simulink library "EV_ePWT"  (R2019b)
settings: Solver=VariableStepAuto  StartTime=0.0  StopTime=10.0  RelTol=1e-3
undefined symbols (not defined in the file): BTR, DiscIntNeverNeededParam, INV
libraries: simulink x1
(part 2 of 2)

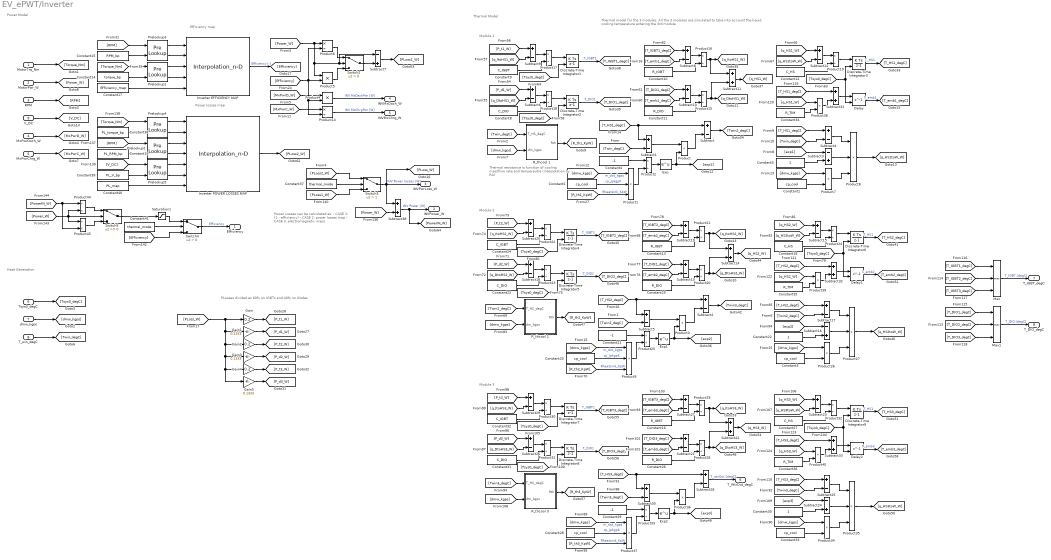
== system EV_ePWT/Inverter ==
  note: Efficiency map
  note: Module 1
  note: Heat Generation
  note: Power Model
  note: Thermal Model
  note: Module 2
  note: Module 3
  note: Power Losses can be calculated as:
      | - CASE 1: (1 - efficiency)
      | - CASE 2: power losses map
      | - CASE 3: electromagnetic maps
  note: PLosses divided as 60% on IGBTs and 40% on diodes
  note: Thermal model for the 3 modules. All the 3 modules are simulated to take into account the liquid cooling temperature entering the 3rd module
  note: Thermal resistance is function of cooling massflow rate and temperautre (interpolation by RA)
  note: Power losses map
  MotorTrq_Nm : Inport
  MotorPwr_W : Inport  Port=2
  RPM : Inport  Port=3
  MxPwrDsch_W : Inport  Port=4
  MxPwrChrg_W : Inport  Port=5
  Tsys0_degC : Inport  Port=6
  dmw_kgps : Inport  Port=7
  T_win_degC : Inport  Port=8
  V_DC : Inport  Port=9
  Constant{1..3,20,28,33} (6 alike) : Constant  Value=cp_cool
  Constant10 : Constant  Value=R_IGBT
  Constant11 : Constant  Value=R_DIO
  Constant12 : Constant  Value=C_HS
  Constant13 : Constant  Value=R_IGBT
  Constant14 : Constant  Value=torque_bp
  Constant15 : Constant  Value=RPM_bp
  Constant16 : Constant  Value=R_IGBT
  Constant17 : Constant  Value=Efficiency_map
  Constant18 : Constant  Value=C_HS
  Constant19 : Constant  Value=PL_RPM_bp
  Constant21 : Constant  Value=-1
  Constant22 : Constant
  Constant23 : Constant  Value=C_DIO
  Constant24 : Constant  Value=C_IGBT
  Constant25 : Constant  Value=R_DIO
  Constant26 : Constant  Value=R_DIO
  Constant27 : Constant  Value=C_HS
  Constant29 : Constant  Value=-1
  Constant30 : Constant
  Constant31 : Constant  Value=C_DIO
  Constant32 : Constant  Value=C_IGBT
  Constant34 : Constant  Value=R_TIM
  Constant35 : Constant  Value=R_TIM
  Constant36 : Constant  Value=R_TIM
  Constant37 : Constant  Value=thermal_mode
  Constant38 : Constant  Value=PL_torque_bp
  Constant39 : Constant  Value=PL_V_bp
  Constant4 : Constant  Value=-1
  Constant40 : Constant  Value=PL_map
  Constant41 : Constant  Value=thermal_mode
  Constant5 : Constant
  Constant8 : Constant  Value=C_DIO
  Constant9 : Constant  Value=C_IGBT
  Delay : Delay  DelayLength=1  InitialConditionSource=Input port
      settings: InputPortMap=u0,p4
  Delay1 : Delay  DelayLength=1  InitialConditionSource=Input port
      settings: InputPortMap=u0,p4
  Delay2 : Delay  DelayLength=1  InitialConditionSource=Input port
      settings: InputPortMap=u0,p4
  Discrete-Time Integrator{1..9} (9 alike) : DiscreteIntegrator  InitialConditionSource=external  SampleTime=-1  ICPrevOutput=DiscIntNeverNeededParam  ICPrevScaledInput=DiscIntNeverNeededParam
  Exp : Math  SaturateOnIntegerOverflow=on
  Exp1 : Math  SaturateOnIntegerOverflow=on
  Exp2 : Math  SaturateOnIntegerOverflow=on
  Gain : Gain  Gain=0.2
  Gain1 : Gain  Gain=0.1333
  Gain2 : Gain  Gain=0.2
  Gain3 : Gain  Gain=0.1333
  Gain4 : Gain  Gain=0.2
  Gain5 : Gain  Gain=0.1333
  Inverter EFFICIENCY MAP : Interpolation_n-D  TableSource=Input port
      settings: InputPortMap=u0,u1,u2,u3,p2
  Inverter POWER LOSSES MAP : Interpolation_n-D  NumberOfTableDimensions=3  TableSource=Input port
      settings: InputPortMap=u0,u1,u2,u3,u4,u5,p2
  Max : MinMax  Function=max  Inputs=3
  Max1 : MinMax  Function=max  Inputs=3
  Prelookup{1..5} (5 alike) : PreLookup  BreakpointsDataSource=Input port  BreakpointsData=[1:4]  ExtrapMethod=Linear  FractionDataTypeStr=double
      settings: InputPortMap=u0,p1
  Product{,3..5,7,26,34,36} (8 alike) : Product
  Product{1,8..9,27,35,37} (6 alike) : Product  Inputs=3
  Product{2,6,14..25,28..33} (20 alike) : Product  Inputs=*/
  Product38 : Product  Inputs=**
  Product39 : Product  Inputs=**
  Product40 : Product  Inputs=**
  Product44 : Product  Inputs=/*
  Product45 : Product  Inputs=/*
  R_thcool 1 : MATLAB Function  TreatAsAtomicUnit=on
  R_thcool 2 : MATLAB Function  TreatAsAtomicUnit=on
  R_thcool 3 : MATLAB Function  TreatAsAtomicUnit=on
  Saturation1 : Saturate  UpperLimit=1  LowerLimit=0.25
  Subtract{,1..2,4..6,8..10,12..13,15,17..21,23,25..30} (24 alike) : Sum  Inputs=+-
  Subtract{11,14,22,31..33,38} (7 alike) : Sum
  Subtract{3,7,16,24} (4 alike) : Sum  Inputs=-+
  Switch2 : Switch  Criteria=u2 > Threshold
  Switch3 : Switch  Criteria=u2 > Threshold  Threshold=1
  Switch4 : Switch  Criteria=u2 > Threshold
  Switch5 : Switch
  Efficiency : Outport
  INVPower_W : Outport  Port=2
  INVPwrLoss_W : Outport  Port=3
  INVMxDsch_W : Outport  Port=4
  INVMxChrg_W : Outport  Port=5
  T_WtrOut_degC : Outport  Port=6
  T_IGBT_degC : Outport  Port=7
  T_DIO_degC : Outport  Port=8
  wires:
  Delay2/1 -> [T_emb3_degC]  "T_emb3"
  Subtract33/1 -> Delay2/1
  Product40/1 -> Subtract33/2
  [T_HS3_degC] -> Subtract33/1
  Constant36/1 -> Product40/2
  [q_HS3_W] -> Product40/1
  [Tsys0_degC] -> Discrete-Time Integrator9/2, Delay2/2
  [Tsys0_degC] -> Discrete-Time Integrator6/2, Delay1/2
  [q_HS2_W] -> Product39/1
  Constant35/1 -> Product39/2
  [T_HS2_degC] -> Subtract32/1
  Product39/1 -> Subtract32/2
  Subtract32/1 -> Delay1/1
  Delay1/1 -> [T_emb2_degC]  "T_emb2"
  Delay/1 -> [T_emb1_degC]  "T_emb1"
  Subtract31/1 -> Delay/1
  Product38/1 -> Subtract31/2
  [T_HS1_degC] -> Subtract31/1
  Constant34/1 -> Product38/2
  [q_HS1_W] -> Product38/1
  R_thcool 1/1(Rth) -> [R_th1_KpW]
  T_win_degC/1 -> [Twin_degC]
  dmw_kgps/1 -> [dmw_kgps]
  Product6/1 -> Switch2/1
  [Efficiency] -> Product5/2, Product6/2, Product14/2, Product4/2
  [RPM] -> Prelookup3/1
  Prelookup3/1 -> Inverter EFFICIENCY MAP/1
  Prelookup3/2 -> Inverter EFFICIENCY MAP/2
  Constant15/1 -> Prelookup3/2
  Inverter EFFICIENCY MAP/1 -> [Efficiency]  "Efficiency [-]"
  MotorTrq_Nm/1 -> [Torque_Nm]
  Tsys0_degC/1 -> [Tsys0_degC]
  MxPwrDsch_W/1 -> [MxPwrD_W]
  RPM/1 -> [RPM]
  MxPwrChrg_W/1 -> [MxPwrC_W]
  MotorPwr_W/1 -> [Power_W]
  [Power_W] -> Subtract7/1, Switch2/2, Product5/1, Product6/1
  [MxPwrD_W] -> Product4/1
  Product4/1 -> INVMxDsch_W/1  "INV MxDschPwr [W]"
  Product14/1 -> INVMxChrg_W/1  "INV MxChrgPwr [W]"
  [MxPwrC_W] -> Product14/1
  Subtract4/1 -> Product8/1
  Product8/1 -> [q_HS1toW_W]
  [dmw_kgps] -> Product1/1  "m_dot_kgps"
  Product7/1 -> Product8/3
  Subtract1/1 -> Product/1
  [T_HS1_degC] -> Subtract4/1
  [dmw_kgps] -> Product7/1
  [Twin_degC] -> Subtract4/2
  Subtract3/1 -> Product8/2
  Product/1 -> Subtract/2
  Exp/1 -> [exp1], Product/2
  Constant2/1 -> Product1/2  "cp_JpkgpK"
  Constant1/1 -> Product7/2
  [R_th1_KpW] -> Product1/3  "Rheatsink_KpW"
  Product2/1 -> Exp/1
  Product1/1 -> Product2/2
  Constant4/1 -> Product2/1
  [Twin_degC] -> Subtract1/2
  [T_HS1_degC] -> Subtract1/1, Subtract/1
  [exp1] -> Subtract3/1
  Constant5/1 -> Subtract3/2
  V_DC/1 -> [V_DC]
  Subtract9/1 -> Product17/1
  [q_DtoHS1_W] -> Subtract6/2
  Discrete-Time Integrator1/1 -> [T_IGBT1_degC]  "T_IGBT1"
  Constant8/1 -> Product18/2
  Subtract6/1 -> Product18/1
  Product18/1 -> Discrete-Time Integrator2/1
  [Tsys0_degC] -> Discrete-Time Integrator2/2
  [P_t1_W] -> Subtract9/1
  Subtract11/1 -> [q_HS1_W]
  [P_d1_W] -> Subtract6/1
  Product17/1 -> Discrete-Time Integrator1/1
  Discrete-Time Integrator2/1 -> [T_DIO1_degC]  "T_DIO1"
  [Tsys0_degC] -> Discrete-Time Integrator1/2
  [q_ItoHS1_W] -> Subtract9/2
  Constant9/1 -> Product17/2
  Subtract8/1 -> Product16/1
  [T_IGBT1_degC] -> Subtract8/1
  [T_emb1_degC] -> Subtract8/2
  Constant10/1 -> Product16/2
  Constant11/1 -> Product15/2
  [T_emb1_degC] -> Subtract10/2
  [T_DIO1_degC] -> Subtract10/1
  Subtract10/1 -> Product15/1
  Product16/1 -> Subtract11/1, [q_ItoHS1_W]
  Product15/1 -> Subtract11/2, [q_DtoHS1_W]
  Constant12/1 -> Product19/2
  [Tsys0_degC] -> Discrete-Time Integrator3/2, Delay/2
  Product19/1 -> Discrete-Time Integrator3/1
  Subtract12/1 -> Product19/1
  [q_HS1_W] -> Subtract12/1
  [q_HS1toW_W] -> Subtract12/2
  Discrete-Time Integrator3/1 -> [T_HS1_degC]  "T_HS1"
  [Twin_degC] -> R_thcool 1/1(T_HS_degC)
  [dmw_kgps] -> R_thcool 1/2(dm_kgps)
  Subtract/1 -> [Twin2_degC]
  Subtract2/1 -> [Twin3_degC]
  R_thcool 2/1(Rth) -> [R_th2_KpW]
  [dmw_kgps] -> R_thcool 2/2(dm_kgps)
  [Twin2_degC] -> R_thcool 2/1(T_HS_degC)
  Discrete-Time Integrator6/1 -> [T_HS2_degC]  "T_HS1"
  [q_HS2toW_W] -> Subtract15/2
  [q_HS2_W] -> Subtract15/1
  Subtract15/1 -> Product24/1
  Product24/1 -> Discrete-Time Integrator6/1
  Constant18/1 -> Product24/2
  Product20/1 -> [q_DtoHS2_W], Subtract14/2
  Product21/1 -> [q_ItoHS2_W], Subtract14/1
  Subtract13/1 -> Product20/1
  [T_DIO2_degC] -> Subtract13/1
  [T_emb2_degC] -> Subtract13/2
  Constant25/1 -> Product20/2
  Constant13/1 -> Product21/2
  [T_emb2_degC] -> Subtract19/2
  [T_IGBT2_degC] -> Subtract19/1
  Subtract19/1 -> Product21/1
  Constant24/1 -> Product22/2
  [q_ItoHS2_W] -> Subtract20/2
  [Tsys0_degC] -> Discrete-Time Integrator4/2
  Discrete-Time Integrator5/1 -> [T_DIO2_degC]  "T_DIO1"
  Product22/1 -> Discrete-Time Integrator4/1
  [P_d2_W] -> Subtract18/1
  Subtract14/1 -> [q_HS2_W]
  [P_t2_W] -> Subtract20/1
  [Tsys0_degC] -> Discrete-Time Integrator5/2
  Product23/1 -> Discrete-Time Integrator5/1
  Subtract18/1 -> Product23/1
  Constant23/1 -> Product23/2
  Discrete-Time Integrator4/1 -> [T_IGBT2_degC]  "T_IGBT1"
  [q_DtoHS2_W] -> Subtract18/2
  Subtract20/1 -> Product22/1
  Constant22/1 -> Subtract16/2
  [exp2] -> Subtract16/1
  [T_HS2_degC] -> Subtract2/1, Subtract5/1
  [Twin2_degC] -> Subtract5/2
  Constant21/1 -> Product25/1
  Product9/1 -> Product25/2
  Product25/1 -> Exp1/1
  [R_th2_KpW] -> Product9/3  "Rheatsink_KpW"
  Constant3/1 -> Product26/2
  Constant20/1 -> Product9/2  "cp_JpkgpK"
  Exp1/1 -> Product3/2, [exp2]
  Product3/1 -> Subtract2/2
  Subtract16/1 -> Product27/2
  [Twin2_degC] -> Subtract17/2
  [dmw_kgps] -> Product26/1
  [T_HS2_degC] -> Subtract17/1
  Subtract5/1 -> Product3/1
  Product26/1 -> Product27/3
  [dmw_kgps] -> Product9/1  "m_dot_kgps"
  Product27/1 -> [q_HS2toW_W]
  Subtract17/1 -> Product27/1
  Subtract25/1 -> Product35/1
  Product35/1 -> [q_HS3toW_W]
  [dmw_kgps] -> Product37/1  "m_dot_kgps"
  Product34/1 -> Product35/3
  Subtract30/1 -> Product36/1
  [T_HS3_degC] -> Subtract25/1
  [dmw_kgps] -> Product34/1
  [Twin3_degC] -> Subtract25/2
  Subtract24/1 -> Product35/2
  Product36/1 -> Subtract28/2
  Exp2/1 -> [exp3], Product36/2
  Constant28/1 -> Product37/2  "cp_JpkgpK"
  Constant33/1 -> Product34/2
  [R_th3_KpW] -> Product37/3  "Rheatsink_KpW"
  Product33/1 -> Exp2/1
  Product37/1 -> Product33/2
  Constant29/1 -> Product33/1
  [Twin3_degC] -> Subtract30/2
  [T_HS3_degC] -> Subtract30/1, Subtract28/1
  [exp3] -> Subtract24/1
  Constant30/1 -> Subtract24/2
  Subtract29/1 -> Product30/1
  [q_DtoHS3_W] -> Subtract26/2
  Discrete-Time Integrator7/1 -> [T_IGBT3_degC]  "T_IGBT1"
  Constant31/1 -> Product31/2
  Subtract26/1 -> Product31/1
  Product31/1 -> Discrete-Time Integrator8/1
  [Tsys0_degC] -> Discrete-Time Integrator8/2
  [P_t3_W] -> Subtract29/1
  Subtract22/1 -> [q_HS3_W]
  [P_d3_W] -> Subtract26/1
  Product30/1 -> Discrete-Time Integrator7/1
  Discrete-Time Integrator8/1 -> [T_DIO3_degC]  "T_DIO1"
  [Tsys0_degC] -> Discrete-Time Integrator7/2
  [q_ItoHS3_W] -> Subtract29/2
  Constant32/1 -> Product30/2
  Subtract27/1 -> Product29/1
  [T_IGBT3_degC] -> Subtract27/1
  [T_emb3_degC] -> Subtract27/2
  Constant16/1 -> Product29/2
  Constant26/1 -> Product28/2
  [T_emb3_degC] -> Subtract21/2
  [T_DIO3_degC] -> Subtract21/1
  Subtract21/1 -> Product28/1
  Product29/1 -> Subtract22/1, [q_ItoHS3_W]
  Product28/1 -> Subtract22/2, [q_DtoHS3_W]
  Constant27/1 -> Product32/2
  Product32/1 -> Discrete-Time Integrator9/1
  Subtract23/1 -> Product32/1
  [q_HS3_W] -> Subtract23/1
  [q_HS3toW_W] -> Subtract23/2
  Discrete-Time Integrator9/1 -> [T_HS3_degC]  "T_HS1"
  [Twin3_degC] -> R_thcool 3/1(T_HS_degC)
  [dmw_kgps] -> R_thcool 3/2(dm_kgps)
  R_thcool 3/1(Rth) -> [R_th3_KpW]
  Subtract28/1 -> T_WtrOut_degC/1  "T_wtrOut [degC]"
  Max/1 -> T_IGBT_degC/1  "T_IGBT [degC]"
  Max1/1 -> T_DIO_degC/1  "T_DIO [degC]"
  Product5/1 -> Switch2/3
  Switch2/1 -> Subtract7/2
  [Power_W] -> Subtract38/2
  Subtract38/1 -> [PowerIN_W], INVPower_W/1  "INV Power [W]"
  Prelookup1/2 -> Inverter EFFICIENCY MAP/4
  Prelookup1/1 -> Inverter EFFICIENCY MAP/3
  [Torque_Nm] -> Prelookup1/1
  Constant14/1 -> Prelookup1/2
  Constant17/1 -> Inverter EFFICIENCY MAP/5
  Constant19/1 -> Prelookup2/2
  Constant38/1 -> Prelookup4/2
  Prelookup4/1 -> Inverter POWER LOSSES MAP/1
  Prelookup4/2 -> Inverter POWER LOSSES MAP/2
  Prelookup2/1 -> Inverter POWER LOSSES MAP/3
  Prelookup2/2 -> Inverter POWER LOSSES MAP/4
  Constant39/1 -> Prelookup5/2
  Prelookup5/2 -> Inverter POWER LOSSES MAP/6
  Prelookup5/1 -> Inverter POWER LOSSES MAP/5
  [V_DC] -> Prelookup5/1
  [Torque_Nm] -> Prelookup4/1
  [RPM] -> Prelookup2/1
  Constant40/1 -> Inverter POWER LOSSES MAP/7
  Inverter POWER LOSSES MAP/1 -> [PLoss2_W]
  Subtract7/1 -> [PLoss1_W]
  [PLoss2_W] -> Switch3/1
  Constant37/1 -> Switch3/2
  Switch3/1 -> [PLoss_W], Subtract38/1, INVPwrLoss_W/1  "INV Power losses [W]"
  [PowerIN_W] -> Product45/2, Product44/1
  Product44/1 -> Switch5/1
  Product45/1 -> Switch5/3
  [Power_W] -> Product45/1, Product44/2, Switch5/2
  [Efficiency] -> Switch4/3
  Saturation1/1 -> Switch4/1
  Switch4/1 -> Efficiency/1  "Efficiency"
  Constant41/1 -> Switch4/2
  Switch5/1 -> Saturation1/1
  [PLoss1_W] -> Switch3/3
  [PLoss_W] -> Gain5/1, Gain4/1, Gain3/1, Gain2/1, Gain1/1, Gain/1
  [T_IGBT1_degC] -> Max/1
  [T_IGBT2_degC] -> Max/2
  [T_IGBT3_degC] -> Max/3
  [T_DIO1_degC] -> Max1/1
  [T_DIO2_degC] -> Max1/2
  [T_DIO3_degC] -> Max1/3
  Gain/1 -> [P_t1_W]
  Gain2/1 -> [P_t2_W]
  Gain4/1 -> [P_t3_W]
  Gain5/1 -> [P_d3_W]
  Gain3/1 -> [P_d2_W]
  Gain1/1 -> [P_d1_W]

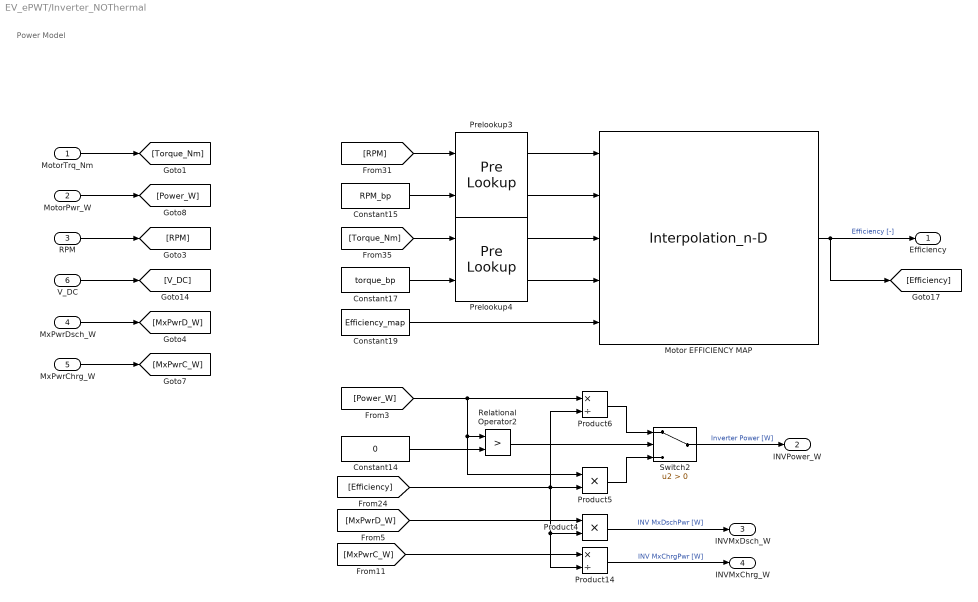
== system EV_ePWT/Inverter_NOThermal ==
  note: Power Model
  MotorTrq_Nm : Inport
  MotorPwr_W : Inport  Port=2
  RPM : Inport  Port=3
  MxPwrDsch_W : Inport  Port=4
  MxPwrChrg_W : Inport  Port=5
  V_DC : Inport  Port=6
  Constant14 : Constant  Value=0
  Constant15 : Constant  Value=RPM_bp
  Constant17 : Constant  Value=torque_bp
  Constant19 : Constant  Value=Efficiency_map
  Motor EFFICIENCY MAP : Interpolation_n-D  TableSource=Input port
      settings: InputPortMap=u0,u1,u2,u3,p2
  Prelookup3 : PreLookup  BreakpointsDataSource=Input port  BreakpointsData=[1:4]  ExtrapMethod=Linear  FractionDataTypeStr=double
      settings: InputPortMap=u0,p1
  Prelookup4 : PreLookup  BreakpointsDataSource=Input port  BreakpointsData=[1:4]  ExtrapMethod=Linear  FractionDataTypeStr=double
      settings: InputPortMap=u0,p1
  Product14 : Product  Inputs=*/
  Product4 : Product
  Product5 : Product
  Product6 : Product  Inputs=*/
  Relational Operator2 : RelationalOperator  Operator=>  OutDataTypeStr=boolean  RndMeth=Simplest
  Switch2 : Switch  Criteria=u2 > Threshold
  Efficiency : Outport
  INVPower_W : Outport  Port=2
  INVMxDsch_W : Outport  Port=3
  INVMxChrg_W : Outport  Port=4
  wires:
  V_DC/1 -> [V_DC]
  [MxPwrC_W] -> Product14/1
  Product14/1 -> INVMxChrg_W/1  "INV MxChrgPwr [W]"
  Product4/1 -> INVMxDsch_W/1  "INV MxDschPwr [W]"
  [MxPwrD_W] -> Product4/1
  [Power_W] -> Product6/1, Relational Operator2/1, Product5/1
  MotorPwr_W/1 -> [Power_W]
  MxPwrChrg_W/1 -> [MxPwrC_W]
  RPM/1 -> [RPM]
  MxPwrDsch_W/1 -> [MxPwrD_W]
  MotorTrq_Nm/1 -> [Torque_Nm]
  Motor EFFICIENCY MAP/1 -> [Efficiency], Efficiency/1  "Efficiency [-]"
  Constant15/1 -> Prelookup3/2
  Prelookup3/2 -> Motor EFFICIENCY MAP/2
  Prelookup4/1 -> Motor EFFICIENCY MAP/3
  Prelookup4/2 -> Motor EFFICIENCY MAP/4
  [Torque_Nm] -> Prelookup4/1
  Prelookup3/1 -> Motor EFFICIENCY MAP/1
  [RPM] -> Prelookup3/1
  Constant17/1 -> Prelookup4/2
  Constant19/1 -> Motor EFFICIENCY MAP/5
  Constant14/1 -> Relational Operator2/2
  Relational Operator2/1 -> Switch2/2
  [Efficiency] -> Product5/2, Product6/2, Product4/2, Product14/2
  Product5/1 -> Switch2/3
  Product6/1 -> Switch2/1
  Switch2/1 -> INVPower_W/1  "Inverter Power [W]"

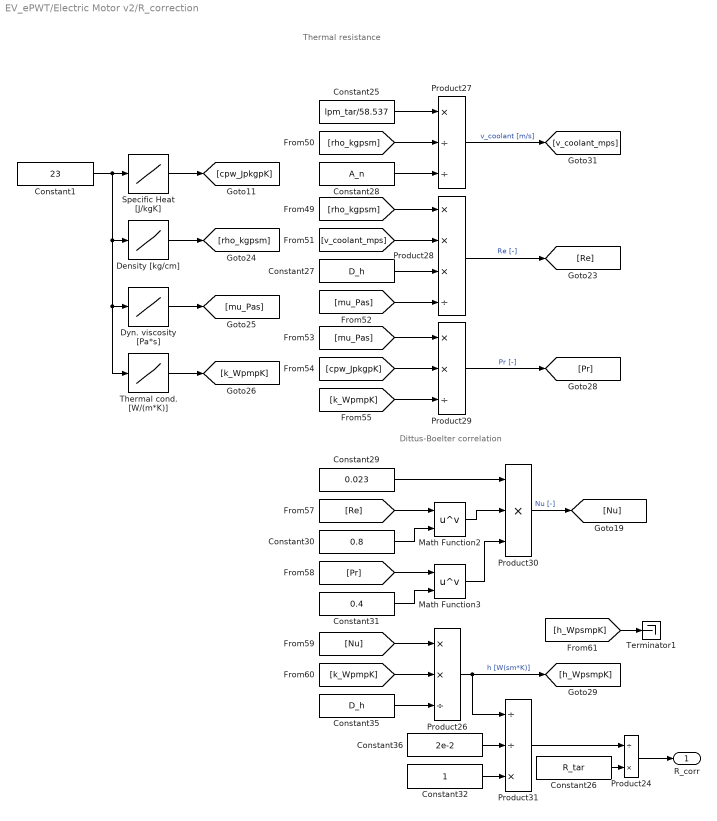
== system EV_ePWT/Electric Motor v2/R_correction ==
  note: Thermal resistance
  note: Dittus-Boelter correlation
  Constant1 : Constant  Value=23
  Constant25 : Constant  Value=lpm_tar/58.537
  Constant26 : Constant  Value=R_tar
  Constant27 : Constant  Value=D_h
  Constant28 : Constant  Value=A_n
  Constant29 : Constant  Value=0.023
  Constant30 : Constant  Value=0.8
  Constant31 : Constant  Value=0.4
  Constant32 : Constant
  Constant35 : Constant  Value=D_h
  Constant36 : Constant  Value=2e-2
  Density [kg/cm] : Lookup_n-D  NumberOfTableDimensions=1  BreakpointsForDimension1=[-45.56 -17.78 10 37.77 65.55 93.33 121.11 148.88 176.66]  Table=[1020,1030,1030,1020,999,985,963,938,911]  ExtrapMethod=Clip  RndMeth=Simplest  InputSameDT=on
  Dyn. viscosity [Pa*s] : Lookup_n-D  NumberOfTableDimensions=1  BreakpointsForDimension1=[-45.56 -17.78 10 37.77 65.55 93.33 121.11 148.88 176.66]  Table=[640.26859,77.622,21.382,10.4477,6.2445,4.2234,3.1074,2.4377,1.98204]*1e-04  ExtrapMethod=Clip  RndMeth=Simplest  InputSameDT=on
  Math Function2 : Math  Operator=pow  SaturateOnIntegerOverflow=on
  Math Function3 : Math  Operator=pow  SaturateOnIntegerOverflow=on
  Product24 : Product  Inputs=/*
  Product26 : Product  Inputs=**/
  Product27 : Product  Inputs=*//
  Product28 : Product  Inputs=***/
  Product29 : Product  Inputs=**/
  Product30 : Product  Inputs=***
  Product31 : Product  Inputs=//*
  Specific Heat [J/kgK] : Lookup_n-D  NumberOfTableDimensions=1  BreakpointsForDimension1=[-45.56 -17.78 10 37.77 65.55 93.33 121.11 148.88 176.66]  Table=[3841.6,3888.1,3934.6,3981.1,4027.6,4074.0,4120.5,4167.0,4213.6]  ExtrapMethod=Clip  RndMeth=Simplest  InputSameDT=on
  Terminator1 : Terminator
  Thermal cond. [W/(m*K)] : Lookup_n-D  NumberOfTableDimensions=1  BreakpointsForDimension1=[-45.56 -17.78 10 37.77 65.55 93.33 121.11 148.88 176.66]  Table=[0.433474,0.474305,0.507306,0.532476,0.549815,0.559304,0.561011,0.554885,0.540929]  ExtrapMethod=Clip  RndMeth=Simplest  InputSameDT=on
  R_corr : Outport
  wires:
  [k_WpmpK] -> Product29/3
  [mu_Pas] -> Product29/1
  Product27/1 -> [v_coolant_mps]  "v_coolant [m/s]"
  [Nu] -> Product26/1
  Product29/1 -> [Pr]  "Pr [-]"
  [cpw_JpkgpK] -> Product29/2
  Product28/1 -> [Re]  "Re [-]"
  [Re] -> Math Function2/1
  [rho_kgpsm] -> Product28/1
  [mu_Pas] -> Product28/4
  [v_coolant_mps] -> Product28/2
  Constant32/1 -> Product31/3
  [Pr] -> Math Function3/1
  Constant27/1 -> Product28/3
  Constant28/1 -> Product27/3
  [rho_kgpsm] -> Product27/2
  Constant30/1 -> Math Function2/2
  [h_WpsmpK] -> Terminator1/1
  Constant36/1 -> Product31/2
  Product26/1 -> Product31/1, [h_WpsmpK]  "h [W(sm*K)]"
  Constant35/1 -> Product26/3
  [k_WpmpK] -> Product26/2
  Product30/1 -> [Nu]  "Nu [-]"
  Math Function3/1 -> Product30/3
  Math Function2/1 -> Product30/2
  Constant31/1 -> Math Function3/2
  Constant29/1 -> Product30/1
  Density [kg/cm]/1 -> [rho_kgpsm]
  Dyn. viscosity [Pa*s]/1 -> [mu_Pas]
  Specific Heat [J/kgK]/1 -> [cpw_JpkgpK]
  Thermal cond. [W/(m*K)]/1 -> [k_WpmpK]
  Constant1/1 -> Density [kg/cm]/1, Thermal cond. [W/(m*K)]/1, Dyn. viscosity [Pa*s]/1, Specific Heat [J/kgK]/1
  Constant25/1 -> Product27/1
  Constant26/1 -> Product24/2
  Product24/1 -> R_corr/1
  Product31/1 -> Product24/1

== matlab function EV_ePWT/Inverter/R_thcool 1 ==
  data: T_HS_degC input; Rth output; dm_kgps input
function Rth = R_thcool(T_HS_degC,dm_kgps)

dm_kgps     = dm_kgps*60;
if dm_kgps > 30
    dm_kgps = 30;
elseif dm_kgps < 1
    dm_kgps = 1;
end
if T_HS_degC > 100
    T_HS_degC = 100;
elseif T_HS_degC < 20
    T_HS_degC = 20;
end

p00 =     0.04335; %  (0.03758, 0.04912)
p10 =   9.341e-05; %  (-0.000112, 0.0002988)
p01 =   -0.004983; %  (-0.007523, -0.002443)
p20 =  -6.834e-07; %  (-2.346e-06, 9.795e-07)
p11 =  -8.584e-05; %  (-0.0001525, -1.922e-05)
p02 =   0.0004813; %  (8.913e-05, 0.0008734)
p21 =   2.522e-07; %  (-2.612e-07, 7.656e-07)
p12 =   7.406e-06; %  (1.49e-06, 1.332e-05)
p03 =  -3.151e-05; %  (-6.007e-05, -2.953e-06)
p22 =  -1.022e-08; %  (-4.989e-08, 2.946e-08)
p13 =   -2.47e-07; %  (-4.474e-07, -4.647e-08)
p04 =   1.028e-06; %  (5.091e-08, 2.005e-06)
p23 =   8.794e-11; %  (-7.521e-10, 9.28e-10)
p14 =    3.03e-09; %  (2.526e-10, 5.808e-09)
p05 =  -1.255e-08; %  (-2.505e-08, -4.493e-11)

Rth   = p00 + p10*T_HS_degC + p01*dm_kgps + p20*T_HS_degC^2 + p11*T_HS_degC*dm_kgps + p02*dm_kgps^2 + p21*T_HS_degC^2*dm_kgps + ...
        p12*T_HS_degC*dm_kgps^2 + p03*dm_kgps^3 + p22*T_HS_degC^2*dm_kgps^2 + p13*T_HS_degC*dm_kgps^3 + p04*dm_kgps^4 + ...
        p23*T_HS_degC^2*dm_kgps^3 + p14*T_HS_degC*dm_kgps^4 + p05*dm_kgps^5 + 0.005;
end

== matlab function EV_ePWT/Inverter/R_thcool 2 ==
  data: T_HS_degC input; Rth output; dm_kgps input
function Rth = R_thcool(T_HS_degC,dm_kgps)

dm_kgps     = dm_kgps*60;
if dm_kgps > 30
    dm_kgps = 30;
elseif dm_kgps < 1
    dm_kgps = 1;
end
if T_HS_degC > 100
    T_HS_degC = 100;
elseif T_HS_degC < 20
    T_HS_degC = 20;
end

p00 =     0.04335; %  (0.03758, 0.04912)
p10 =   9.341e-05; %  (-0.000112, 0.0002988)
p01 =   -0.004983; %  (-0.007523, -0.002443)
p20 =  -6.834e-07; %  (-2.346e-06, 9.795e-07)
p11 =  -8.584e-05; %  (-0.0001525, -1.922e-05)
p02 =   0.0004813; %  (8.913e-05, 0.0008734)
p21 =   2.522e-07; %  (-2.612e-07, 7.656e-07)
p12 =   7.406e-06; %  (1.49e-06, 1.332e-05)
p03 =  -3.151e-05; %  (-6.007e-05, -2.953e-06)
p22 =  -1.022e-08; %  (-4.989e-08, 2.946e-08)
p13 =   -2.47e-07; %  (-4.474e-07, -4.647e-08)
p04 =   1.028e-06; %  (5.091e-08, 2.005e-06)
p23 =   8.794e-11; %  (-7.521e-10, 9.28e-10)
p14 =    3.03e-09; %  (2.526e-10, 5.808e-09)
p05 =  -1.255e-08; %  (-2.505e-08, -4.493e-11)

Rth   = p00 + p10*T_HS_degC + p01*dm_kgps + p20*T_HS_degC^2 + p11*T_HS_degC*dm_kgps + p02*dm_kgps^2 + p21*T_HS_degC^2*dm_kgps + ...
        p12*T_HS_degC*dm_kgps^2 + p03*dm_kgps^3 + p22*T_HS_degC^2*dm_kgps^2 + p13*T_HS_degC*dm_kgps^3 + p04*dm_kgps^4 + ...
        p23*T_HS_degC^2*dm_kgps^3 + p14*T_HS_degC*dm_kgps^4 + p05*dm_kgps^5 + 0.005;
end

== matlab function EV_ePWT/Inverter/R_thcool 3 ==
  data: T_HS_degC input; Rth output; dm_kgps input
function Rth = R_thcool(T_HS_degC,dm_kgps)

dm_kgps     = dm_kgps*60;
if dm_kgps > 30
    dm_kgps = 30;
elseif dm_kgps < 1
    dm_kgps = 1;
end
if T_HS_degC > 100
    T_HS_degC = 100;
elseif T_HS_degC < 20
    T_HS_degC = 20;
end

p00 =     0.04335; %  (0.03758, 0.04912)
p10 =   9.341e-05; %  (-0.000112, 0.0002988)
p01 =   -0.004983; %  (-0.007523, -0.002443)
p20 =  -6.834e-07; %  (-2.346e-06, 9.795e-07)
p11 =  -8.584e-05; %  (-0.0001525, -1.922e-05)
p02 =   0.0004813; %  (8.913e-05, 0.0008734)
p21 =   2.522e-07; %  (-2.612e-07, 7.656e-07)
p12 =   7.406e-06; %  (1.49e-06, 1.332e-05)
p03 =  -3.151e-05; %  (-6.007e-05, -2.953e-06)
p22 =  -1.022e-08; %  (-4.989e-08, 2.946e-08)
p13 =   -2.47e-07; %  (-4.474e-07, -4.647e-08)
p04 =   1.028e-06; %  (5.091e-08, 2.005e-06)
p23 =   8.794e-11; %  (-7.521e-10, 9.28e-10)
p14 =    3.03e-09; %  (2.526e-10, 5.808e-09)
p05 =  -1.255e-08; %  (-2.505e-08, -4.493e-11)

Rth   = p00 + p10*T_HS_degC + p01*dm_kgps + p20*T_HS_degC^2 + p11*T_HS_degC*dm_kgps + p02*dm_kgps^2 + p21*T_HS_degC^2*dm_kgps + ...
        p12*T_HS_degC*dm_kgps^2 + p03*dm_kgps^3 + p22*T_HS_degC^2*dm_kgps^2 + p13*T_HS_degC*dm_kgps^3 + p04*dm_kgps^4 + ...
        p23*T_HS_degC^2*dm_kgps^3 + p14*T_HS_degC*dm_kgps^4 + p05*dm_kgps^5 + 0.005;
end
